simulink model "DC_motor_EX5"  (R2022a)
settings: Solver=VariableStepAuto  StartTime=0.0  StopTime=.5  RelTol=1e-3
values from neighbouring files (symbols this model uses):
  Ad = dis_sys.A    [DC_motor.m]
  B_noise = [Bd ones(size(Bd,1),1) Bw]    [DC_motor.m]
  Bd = dis_sys.B    [DC_motor.m]
  Bw = [-0.0085 -0.0006 ... (first row only)    [DC_motor.m]
  Cd = dis_sys.C    [DC_motor.m]
  Cnew = [0 1]    [DC_motor.m]
  D_noise = [Dd zeros(size(Dd,1),1) Dd Dd ]    [DC_motor.m]
  N = 10    [DC_motor.m]
  Pr = P    [DC_motor.m]
  Q = 1000*eye(2)    [DC_motor.m]
  R = R    (= 1)    [DC_motor.m]
  Rk = Qk(1)*1000000    [DC_motor.m]
  Ts = 1e-3    (= 0.001)    [DC_motor.m]
  Vmax = 12    [DC_motor.m]
  Vmin = 0    [DC_motor.m]
  W = [1 ... (first row only)    [DC_motor.m]
  x0 = [I0 n0]'    [DC_motor.m]
  xmax = [Imax,nmax]'    [DC_motor.m]
  xmin = [Imin,nmin]'    [DC_motor.m]
undefined symbols (not defined in the file or in its folder): Discrete, MPC_Constrainte, Time
libraries: simulink x2, ctrlSharedLib x1
settings Model: Creator=Shahin  LastModifiedBy=jj
settings SolverCC: AlgebraicLoopSolver=TrustRegion
settings DataIOCC: ReturnWorkspaceOutputs=off
settings DebuggingCC: UnconnectedInputMsg=warning  UnconnectedOutputMsg=warning  UnconnectedLineMsg=warning  SFMachineParentedDataDiag=warning  ArithmeticOperatorsInVariantConditions=warning
settings SFSimCC: CustomCodeUndefinedFunction=UseInterfaceOnly

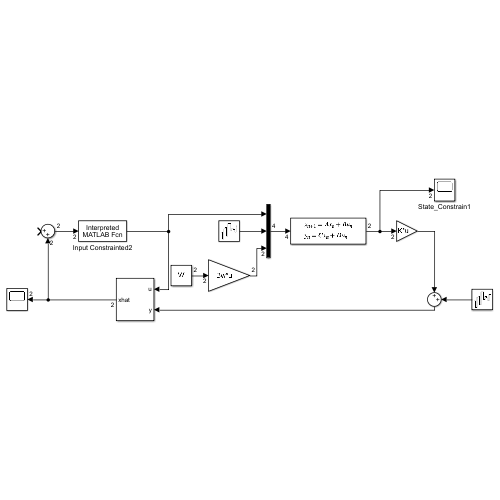
[thumbnail: Simulink's stored preview of the top-level diagram]
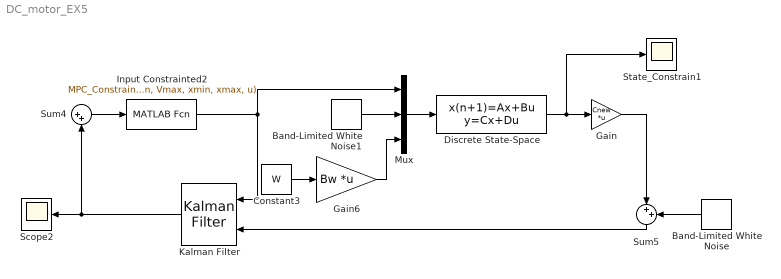
== system DC_motor_EX5 ==
  Band-Limited White Noise : simulink/Sources/Band-Limited White Noise  Cov=power_vy  Ts=Ts  seed=[23341]
  Band-Limited White Noise1 : simulink/Sources/Band-Limited White Noise  Cov=power_vx  Ts=0.1  seed=[2331]
  Constant3 : Constant  Value=W  SampleTime=Ts
  Discrete State-Space : DiscreteStateSpace  A=Ad  B=B_noise  C=Cd  D=D_noise  InitialCondition=x0  SampleTime=Ts
  Gain : Gain  Gain=Cnew  Multiplication=Matrix(K*u)
  Gain6 : Gain  Gain=Bw  Multiplication=Matrix(K*u)
  Input Constrainted2 : MATLABFcn  MATLABFcn=MPC_Constrainte( Ad,Bd, Q, R, Pr, N, Vmin, Vmax, xmin, xmax, u)  OutputDimensions=1
  Kalman Filter : ctrlSharedLib/Kalman Filter  TimeDomain=Discrete-Time  UseCurrentEstimator=on  ModelSource=Individual A, B, C, D matrices  ModelSourceVariable=ss(0.95,1,1,0,1)  A=Ad  B=Bd  C=Cnew  D=0  NumberOfStates=1  NumberOfInputs=1  NumberOfOutputs=1  InitialEstimateSource=Dialog  X0=x0  P0=10  UseK=off  UseGH=off  NumberOfProcessNoiseInputs=1  G=1  TimeInvariantG=on  H=0  TimeInvariantH=on  Q=Qk  TimeInvariantQ=on  R=Rk  TimeInvariantR=on  N=0  TimeInvariantN=on  AddInputPort=on  AddEnablePort=off  OutputEstimatedY=off  OutputP=off  Ts=Ts
  Mux : Mux  Inputs=3
  Scope2 : Scope
  State_Constrain1 : Scope
  Sum4 : Sum  Inputs=|++
  Sum5 : Sum  Inputs=|++
  wires:
  Sum4/1 -> Input Constrainted2/1
  Constant3/1 -> Gain6/1
  Input Constrainted2/1 -> Kalman Filter/1, Mux/1
  Discrete State-Space/1 -> Gain/1, State_Constrain1/1
  Sum5/1 -> Kalman Filter/2
  Band-Limited White Noise/1 -> Sum5/2
  Kalman Filter/1 -> Scope2/1, Sum4/2
  Mux/1 -> Discrete State-Space/1
  Gain6/1 -> Mux/3
  Band-Limited White Noise1/1 -> Mux/2
  Gain/1 -> Sum5/1
